simulink model "dynamic_servers"  (R2019a)
settings: Solver=VariableStepAuto  StartTime=0.0  StopTime=10.0  RelTol=1e-3
undefined symbols (not defined in the file or in its folder): m, n
settings Model: Creator=arsineh  LastModifiedBy=arsineh

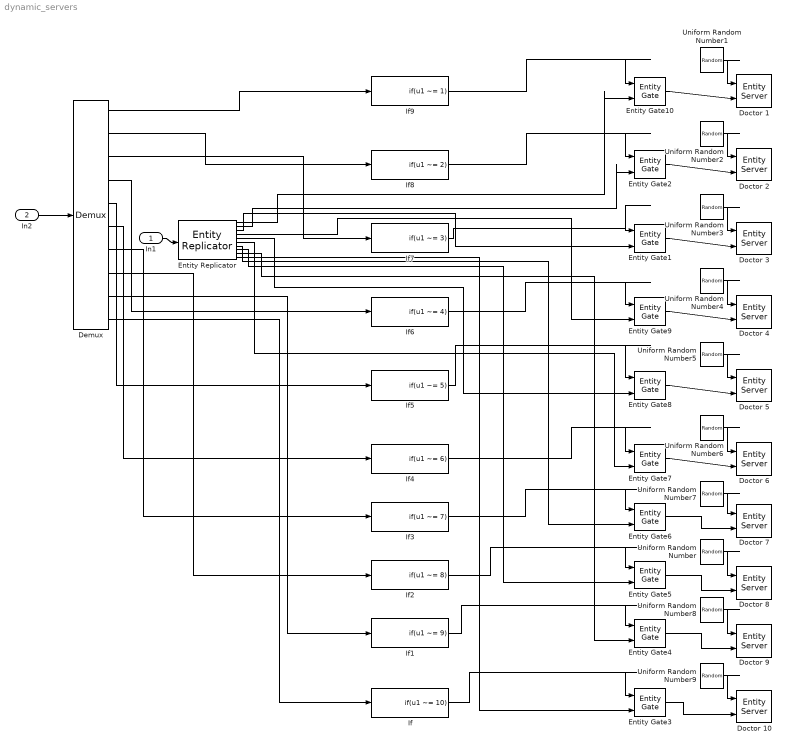
== system dynamic_servers ==
  In1 : Inport
  In2 : Inport  Port=2
  Demux : Demux  Outputs=10
  Doctor 1 : EntityServer  InputPortMessageModes=n,m  OutputPortMessageModes=n,m  Capacity=1  ServiceTimeSource=Signal port  ServiceTimeValue=30  ServiceTimeAction=dt = randi([30,60]);  AverageWait=on
      settings: InputPortMap=u0,u2  OutputPortMap=o4,o9
  Doctor 10 : EntityServer  InputPortMessageModes=n,m  OutputPortMessageModes=n,m  Capacity=10  ServiceTimeSource=Signal port  ServiceTimeValue=30  ServiceTimeAction=dt = randi([30,60]);  AverageWait=on
      settings: InputPortMap=u0,u2  OutputPortMap=o4,o9
  Doctor 2 : EntityServer  InputPortMessageModes=n,m  OutputPortMessageModes=n,m  Capacity=2  ServiceTimeSource=Signal port  ServiceTimeValue=30  ServiceTimeAction=dt = randi([30,60]);  AverageWait=on
      settings: InputPortMap=u0,u2  OutputPortMap=o4,o9
  Doctor 3 : EntityServer  InputPortMessageModes=n,m  OutputPortMessageModes=n,m  Capacity=3  ServiceTimeSource=Signal port  ServiceTimeValue=30  ServiceTimeAction=dt = randi([30,60]);  AverageWait=on
      settings: InputPortMap=u0,u2  OutputPortMap=o4,o9
  Doctor 4 : EntityServer  InputPortMessageModes=n,m  OutputPortMessageModes=n,m  Capacity=4  ServiceTimeSource=Signal port  ServiceTimeValue=30  ServiceTimeAction=dt = randi([30,60]);  AverageWait=on
      settings: InputPortMap=u0,u2  OutputPortMap=o4,o9
  Doctor 5 : EntityServer  InputPortMessageModes=n,m  OutputPortMessageModes=n,m  ServiceTimeSource=Signal port  ServiceTimeValue=30  ServiceTimeAction=dt = randi([30,60]);  AverageWait=on
      settings: InputPortMap=u0,u2  OutputPortMap=o4,o9
  Doctor 6 : EntityServer  InputPortMessageModes=n,m  OutputPortMessageModes=n,m  Capacity=6  ServiceTimeSource=Signal port  ServiceTimeValue=30  ServiceTimeAction=dt = randi([30,60]);  AverageWait=on
      settings: InputPortMap=u0,u2  OutputPortMap=o4,o9
  Doctor 7 : EntityServer  InputPortMessageModes=n,m  OutputPortMessageModes=n,m  Capacity=7  ServiceTimeSource=Signal port  ServiceTimeValue=30  ServiceTimeAction=dt = randi([30,60]);  AverageWait=on
      settings: InputPortMap=u0,u2  OutputPortMap=o4,o9
  Doctor 8 : EntityServer  InputPortMessageModes=n,m  OutputPortMessageModes=n,m  Capacity=8  ServiceTimeSource=Signal port  ServiceTimeValue=30  ServiceTimeAction=dt = randi([30,60]);  AverageWait=on
      settings: InputPortMap=u0,u2  OutputPortMap=o4,o9
  Doctor 9 : EntityServer  InputPortMessageModes=n,m  OutputPortMessageModes=n,m  Capacity=9  ServiceTimeSource=Signal port  ServiceTimeValue=30  ServiceTimeAction=dt = randi([30,60]);  AverageWait=on
      settings: InputPortMap=u0,u2  OutputPortMap=o4,o9
  Entity Gate{1..10} (10 alike) : EntityGate  InputPortMessageModes=m,m  OutputPortMessageModes=m
  Entity Replicator : EntityReplicator  InputPortMessageModes=m  OutputPortMessageModes=m,m,m,m,m,m,m,m,m,m  NumberReplicas=9
      settings: OutputPortMap=o0,o1,o2,o3,o4,o5,o6,o7,o8,o9
  If : If  IfExpression=u1 ~= 10  ShowElse=off
  If1 : If  IfExpression=u1 ~= 9  ShowElse=off
  If2 : If  IfExpression=u1 ~= 8  ShowElse=off
  If3 : If  IfExpression=u1 ~= 7  ShowElse=off
  If4 : If  IfExpression=u1 ~= 6  ShowElse=off
  If5 : If  IfExpression=u1 ~= 5  ShowElse=off
  If6 : If  IfExpression=u1 ~= 4  ShowElse=off
  If7 : If  IfExpression=u1 ~= 3  ShowElse=off
  If8 : If  IfExpression=u1 ~= 2  ShowElse=off
  If9 : If  IfExpression=u1 ~= 1  ShowElse=off
  Uniform Random Number{,1..9} (10 alike) : UniformRandomNumber  Minimum=30  Maximum=60  Seed=234234234  SampleTime=0.1
  wires:
  Uniform Random Number/1 -> Doctor 8/1
  Uniform Random Number1/1 -> Doctor 1/1
  Uniform Random Number2/1 -> Doctor 2/1
  Uniform Random Number3/1 -> Doctor 3/1
  Uniform Random Number4/1 -> Doctor 4/1
  Uniform Random Number5/1 -> Doctor 5/1
  Uniform Random Number6/1 -> Doctor 6/1
  Uniform Random Number7/1 -> Doctor 7/1
  Uniform Random Number8/1 -> Doctor 9/1
  Uniform Random Number9/1 -> Doctor 10/1
  In1/1 -> Entity Replicator/1
  In2/1 -> Demux/1
  Entity Gate2/1 -> Doctor 2/2
  Demux/10 -> If/1
  If/1 -> Entity Gate3/1
  Entity Gate3/1 -> Doctor 10/2
  If1/1 -> Entity Gate4/1
  Entity Gate4/1 -> Doctor 9/2
  Demux/9 -> If1/1
  Demux/8 -> If2/1
  Demux/7 -> If3/1
  Demux/6 -> If4/1
  Demux/5 -> If5/1
  Demux/4 -> If6/1
  Demux/3 -> If7/1
  Demux/2 -> If8/1
  Demux/1 -> If9/1
  Entity Replicator/9 -> Entity Gate4/2
  Entity Replicator/8 -> Entity Gate5/2
  Entity Replicator/7 -> Entity Gate6/2
  Entity Replicator/6 -> Entity Gate7/2
  Entity Replicator/5 -> Entity Gate8/2
  Entity Replicator/4 -> Entity Gate9/2
  Entity Replicator/3 -> Entity Gate1/2
  Entity Replicator/2 -> Entity Gate2/2
  Entity Replicator/10 -> Entity Gate3/2
  Entity Replicator/1 -> Entity Gate10/2
  If2/1 -> Entity Gate5/1
  If3/1 -> Entity Gate6/1
  If4/1 -> Entity Gate7/1
  If5/1 -> Entity Gate8/1
  If6/1 -> Entity Gate9/1
  If7/1 -> Entity Gate1/1
  If8/1 -> Entity Gate2/1
  If9/1 -> Entity Gate10/1
  Entity Gate10/1 -> Doctor 1/2
  Entity Gate1/1 -> Doctor 3/2
  Entity Gate9/1 -> Doctor 4/2
  Entity Gate8/1 -> Doctor 5/2
  Entity Gate7/1 -> Doctor 6/2
  Entity Gate6/1 -> Doctor 7/2
  Entity Gate5/1 -> Doctor 8/2
